simulink model "BBB_Compass_Test_LibraryBlock"  (R2013a)
settings: Solver=FixedStepDiscrete  StartTime=0.0  StopTime=inf  FixedStep=0.01  RelTol=1e-3
libraries: BLACKlink x1
settings Model: SimulationMode=external  ExtModeTrigDuration=100  Creator=rdustinkahawita  LastModifiedBy=rdustinkahawita
settings DataIOCC: InspectSignalLogs=on
settings OptimizationCC: OptimizeModelRefInitCode=on  LifeSpan=1
settings DebuggingCC: SolverPrmCheckMsg=none  StrictBusMsg=Warning
settings HardwareCC: ProdLargestAtomicInteger=Long  ProdLargestAtomicFloat=Double  ProdEndianess=LittleEndian  ProdHWDeviceType=ARM Compatible->ARM Cortex
settings RTWCC: SystemTargetFile=realtime.tlc  GenerateMakefile=off  TemplateMakefile=realtime.tmf  Description=Run on Target Hardware  RTWVerbose=off  ProcessScript=realtime_make_rtw_hook
settings STFCustomTargetCC: TargetLibSuffix=.a  GenerateSampleERTMain=on  ERTCustomFileBanners=on  SupportNonInlinedSFcns=off  SupportVariableSizeSignals=on  MATLABClassNameForMDSCustomization=Simulink.SoftwareTarget.ERTCustomization  SystemTargetFile=realtime.tlc
settings ERTTargetCC: ParMdlRefBuildCompliant=off  CompOptLevelCompliant=off  ConcurrentExecutionCompliant=off  CombineOutputUpdateFcns=off  ERTFirstTimeCompliant=off  SupportContinuousTime=on  SupportVariableSizeSignals=on  ModelStepFunctionPrototypeControlCompliant=off  CPPClassGenCompliant=off  ExtMode=on  ExtModeMexArgs='192.168.7.2' 0 17725  ERTSrcFileBannerTemplate=realtime_code_template.cgt  ERTHdrFileBannerTemplate=realtime_code_template.cgt  ERTDataSrcFileTemplate=realtime_code_template.cgt  ERTDataHdrFileTemplate=realtime_code_template.cgt  ERTCustomFileTemplate=realtime_file_process.tlc

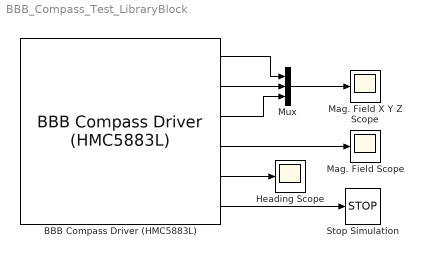
== system BBB_Compass_Test_LibraryBlock ==
  BBB Compass Driver (HMC5883L) : BLACKlink/BBB Compass Driver (HMC5883L)  BBB_I2CBus=BeagleBone Black I2C Channel 1  BBB_I2CAddress=Compass Address: 0x1E  BBB_Compass_DataOutAvrg=1 Sample per Measurement Output  BBB_Compass_DataOutRate=75 Hz  BBB_Compass_MeasureMode=Normal Configuration  BBB_Compass_GainValue=GN3 - Sensor Field Range: +/- 2.50 Ga; Gain: 660 LSb/Gauss  BBB_Compass_OpMode=Continuous Measurement Mode  BBB_Compass_HeadingMode=Output True North  BBB_Compass_HeadingOffset=0  BBB_Compass_DeclinationAng=-14.66  BBB_Compass_SelfTest=on  BBB_Compass_SelfTest_GainValue=GN5 - Sensor Field Range: +/- 4.70 Ga; Gain: 390 LSb/Gauss  BBB_Debug_InfoLevel=No Debug Info
  Heading Scope : Scope
      settings: YMin=0  YMax=375
  Mag. Field Scope : Scope
      settings: YMin=32  YMax=38.5  SaveName=ScopeData2
  Mag. Field X Y Z Scope : Scope
  Mux : Mux  Inputs=3
  Stop Simulation : Stop
  wires:
  BBB Compass Driver (HMC5883L)/6 -> Stop Simulation/1
  BBB Compass Driver (HMC5883L)/5 -> Heading Scope/1
  BBB Compass Driver (HMC5883L)/1 -> Mux/1
  BBB Compass Driver (HMC5883L)/2 -> Mux/2
  BBB Compass Driver (HMC5883L)/3 -> Mux/3
  Mux/1 -> Mag. Field X Y Z Scope/1
  BBB Compass Driver (HMC5883L)/4 -> Mag. Field Scope/1
